simulink model "LAB2"  (R2023a)
settings: Solver=VariableStepAuto  StartTime=0.0  StopTime=10.0  RelTol=1e-3
settings Model: Creator=Mohamed Ezzelrgal  LastModifiedBy=Mohamed Ezzelrgal

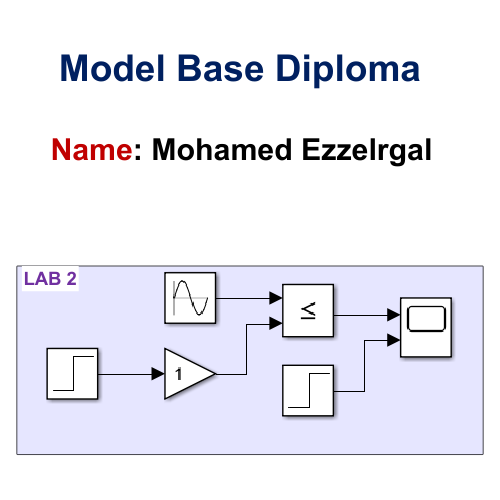
[thumbnail: Simulink's stored preview of the top-level diagram]
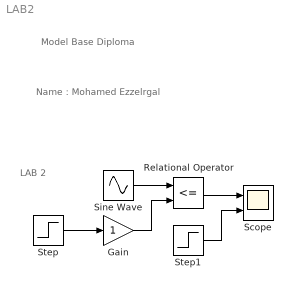
== system LAB2 ==
  note: LAB 2
  note: Model Base Diploma
  note: Name : Mohamed Ezzelrgal
  Gain : Gain
  Relational Operator : RelationalOperator  Operator=<=  OutDataTypeStr=boolean  RndMeth=Simplest  InputSameDT=off
  Scope : Scope  NumInputPorts=2
  Sine Wave : Sin  SampleTime=0
  Step : Step  Time=2  SampleTime=0
  Step1 : Step  Time=2  SampleTime=0
  wires:
  Step/1 -> Gain/1
  Sine Wave/1 -> Relational Operator/1
  Relational Operator/1 -> Scope/1
  Gain/1 -> Relational Operator/2
  Step1/1 -> Scope/2
